simulink library "pathFollowingController_cl"  (R2018b)
settings: Solver=VariableStepAuto  StartTime=0.0  StopTime=10.0  RelTol=1e-3
libraries: filteredPIDController_ul x4, rotationSequence_ul x1, schmehlTangentRotation_ul x1
settings Model: Creator=jldanie5  LastModifiedBy=jldanie5

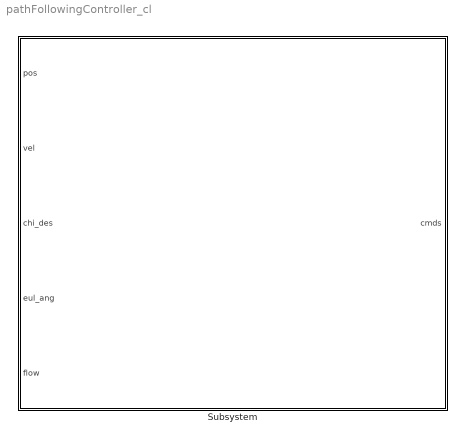
== system pathFollowingController_cl ==
  Subsystem : Subsystem  mask{AoA_des=0}
      mask prompts: AoA_des "Desired Angle of Attack"

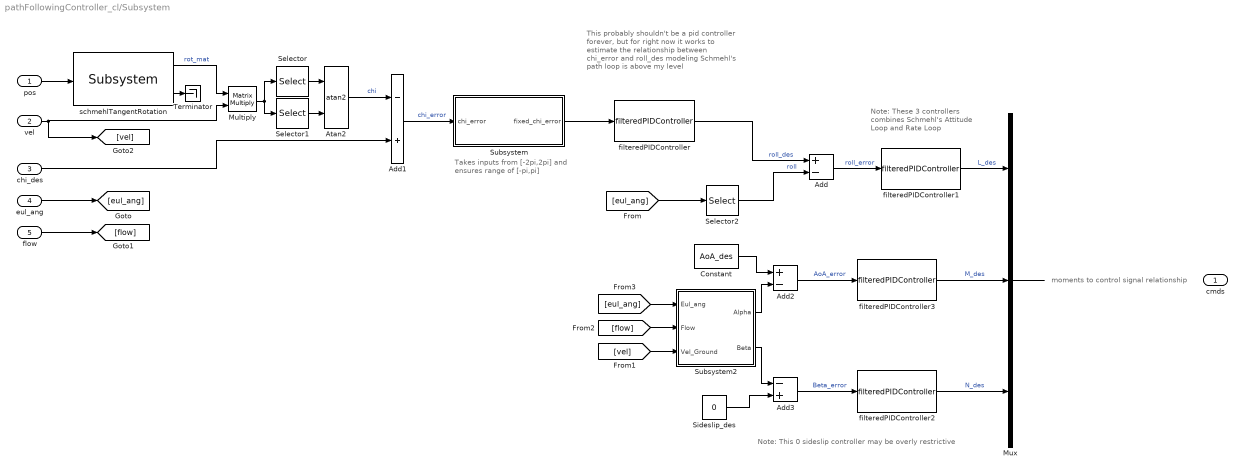
== system pathFollowingController_cl/Subsystem ==
  note: Note: These 3 controllers
      | combines Schmehl's Attitude
      | Loop and Rate Loop
  note: Note: This 0 sideslip controller may be overly restrictive
  note: This probably shouldn't be a pid
      | controller forever, but for right now
      | it works to estimate the relationship
      | between chi_error and roll_des
      |
      | modeling Schmehl's path loop is above
      | my level
  note: Takes inputs from [-2pi,2pi] and
      | ensures range of [-pi,pi]
  note: moments to control signal relationship
  pos : Inport
  vel : Inport  Port=2
  chi_des : Inport  Port=3
  eul_ang : Inport  Port=4
  flow : Inport  Port=5
  Add : Sum  Inputs=+-
  Add1 : Sum  Inputs=-+
  Add2 : Sum  Inputs=+-
  Add3 : Sum  Inputs=-+
  Atan2 : Trigonometry  Operator=atan2
  Constant : Constant  Value=AoA_des
  Multiply : Product  Multiplication=Matrix(*)
  Mux : Mux  Inputs=3
  Selector : Selector  InputPortWidth=3  IndexOptions=Index vector (dialog)  Indices=2  OutputSizes=1
  Selector1 : Selector  InputPortWidth=3  IndexOptions=Index vector (dialog)  Indices=1  OutputSizes=1
  Selector2 : Selector  InputPortWidth=3  IndexOptions=Index vector (dialog)  Indices=1  OutputSizes=1
  Sideslip_des : Constant  Value=0
  Subsystem : Subsystem
  Subsystem2 : Subsystem
  Terminator : Terminator
  filteredPIDController : filteredPIDController_ul/filteredPIDController  kp=kp_chi  ki=kd_chi  kd=0  tau=tau_chi
  filteredPIDController1 : filteredPIDController_ul/filteredPIDController  kp=kp_L  ki=kd_L  kd=0  tau=tau_L
  filteredPIDController2 : filteredPIDController_ul/filteredPIDController  kp=kp_L  ki=kd_L  kd=0  tau=tau_L
  filteredPIDController3 : filteredPIDController_ul/filteredPIDController  kp=kp_M  ki=kd_M  kd=0  tau=tau_M
  schmehlTangentRotation : schmehlTangentRotation_ul/Subsystem  SystemSampleTime=-1
  cmds : Outport
  wires:
  schmehlTangentRotation/2 -> Terminator/1
  schmehlTangentRotation/1 -> Multiply/1  "rot_mat"
  pos/1 -> schmehlTangentRotation/1
  vel/1 -> Multiply/2, [vel]
  Multiply/1 -> Selector/1, Selector1/1
  Selector1/1 -> Atan2/2
  Selector/1 -> Atan2/1
  Atan2/1 -> Add1/1  "chi"
  chi_des/1 -> Add1/2
  [eul_ang] -> Selector2/1
  Selector2/1 -> Add/2  "roll"
  Add/1 -> filteredPIDController1/1  "roll_error"
  filteredPIDController1/1 -> Mux/1  "L_des"
  Mux/1 -> ?
  ? -> cmds/1
  eul_ang/1 -> [eul_ang]
  flow/1 -> [flow]
  Add1/1 -> Subsystem/1(chi_error)  "chi_error"
  Subsystem/1(fixed_chi_error) -> filteredPIDController/1
  filteredPIDController/1 -> Add/1  "roll_des"
  filteredPIDController2/1 -> Mux/3  "N_des"
  filteredPIDController3/1 -> Mux/2  "M_des"
  [eul_ang] -> Subsystem2/1(Eul_ang)
  [flow] -> Subsystem2/2(Flow)
  [vel] -> Subsystem2/3(Vel_Ground)
  Subsystem2/1(Alpha) -> Add2/2
  Constant/1 -> Add2/1
  Add2/1 -> filteredPIDController3/1  "AoA_error"
  Subsystem2/2(Beta) -> Add3/1
  Sideslip_des/1 -> Add3/2
  Add3/1 -> filteredPIDController2/1  "Beta_error"

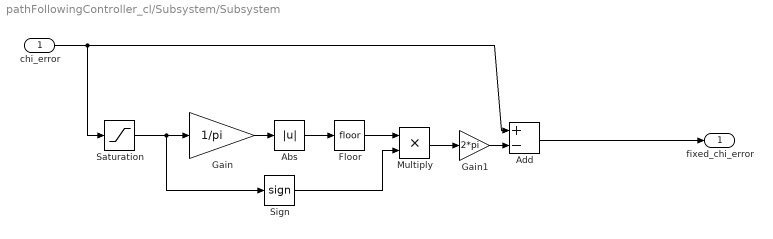
== system pathFollowingController_cl/Subsystem/Subsystem ==
  chi_error : Inport
  Abs : Abs
  Add : Sum  Inputs=+-
  Floor : Rounding
  Gain : Gain  Gain=1/pi
  Gain1 : Gain  Gain=2*pi
  Multiply : Product
  Saturation : Saturate  UpperLimit=pi  LowerLimit=-pi
  Sign : Signum
  fixed_chi_error : Outport
  wires:
  Add/1 -> fixed_chi_error/1
  chi_error/1 -> Saturation/1, Add/1
  Saturation/1 -> Sign/1, Gain/1
  Gain/1 -> Abs/1
  Abs/1 -> Floor/1
  Floor/1 -> Multiply/1
  Sign/1 -> Multiply/2
  Multiply/1 -> Gain1/1
  Gain1/1 -> Add/2

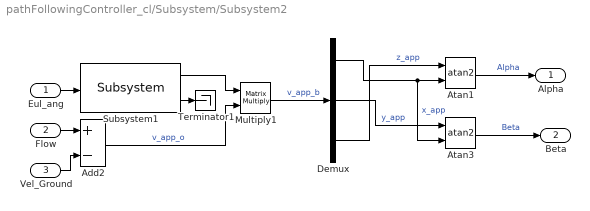
== system pathFollowingController_cl/Subsystem/Subsystem2 ==
  Eul_ang : Inport
  Flow : Inport  Port=2
  Vel_Ground : Inport  Port=3
  Add2 : Sum  Inputs=+-
  Atan1 : Trigonometry  Operator=atan2
  Atan3 : Trigonometry  Operator=atan2
  Demux : Demux  Outputs=3
  Multiply1 : Product  Multiplication=Matrix(*)
  Subsystem1 : rotationSequence_ul/Subsystem  SystemSampleTime=-1
  Terminator1 : Terminator
  Alpha : Outport
  Beta : Outport  Port=2
  wires:
  Demux/1 -> Atan1/2, Atan3/2  "x_app"
  Subsystem1/2 -> Terminator1/1
  Demux/3 -> Atan1/1  "z_app"
  Demux/2 -> Atan3/1  "y_app"
  Subsystem1/1 -> Multiply1/1
  Multiply1/1 -> Demux/1  "v_app_b"
  Eul_ang/1 -> Subsystem1/1
  Add2/1 -> Multiply1/2  "v_app_o"
  Atan3/1 -> Beta/1  "Beta"
  Flow/1 -> Add2/1
  Atan1/1 -> Alpha/1  "Alpha"
  Vel_Ground/1 -> Add2/2
